simulink model "Abraham_PartC1"  (Simulink 9.1)
settings: Solver=VariableStepAuto  StartTime=0.0  StopTime=2  RelTol=1e-3
settings Model: Creator=sophi  LastModifiedBy=sophi
settings SolverCC: ZeroCrossAlgorithm=Adaptive
settings DataIOCC: SaveFormat=Dataset
settings OptimizationCC: LifeSpan=auto
settings DebuggingCC: UnderspecifiedInitializationDetection=Simplified  MergeDetectMultiDrivingBlocksExec=error  MaxConsecutiveZCsMsg=none  SFUnexpectedBacktrackingDiag=error  SFNoUnconditionalDefaultTransitionDiag=error  SFExecutionAtInitializationDiag=warning
settings HardwareCC: ProdBitPerPointer=64  ProdBitPerSizeT=64  ProdBitPerPtrDiffT=64  ProdLargestAtomicFloat=Float  ProdIntDivRoundTo=Zero  ProdEndianess=LittleEndian  ProdWordSize=64  ProdHWDeviceType=Intel->x86-64 (Windows64)
settings ModelReferenceCC: PropagateSignalLabelsOutOfModel=on
settings CodeAppCC: StateflowObjectComments=off
settings GRTTargetCC: TargetLangStandard=C99 (ISO)  CombineOutputUpdateFcns=on  GRTInterface=off
settings ConfigComp: CovMetricSettings=dwe  CovHtmlReporting=off  CovSaveCumulativeToWorkspaceVar=off  CovSaveSingleToWorkspaceVar=off  CovExternalEMLEnable=on

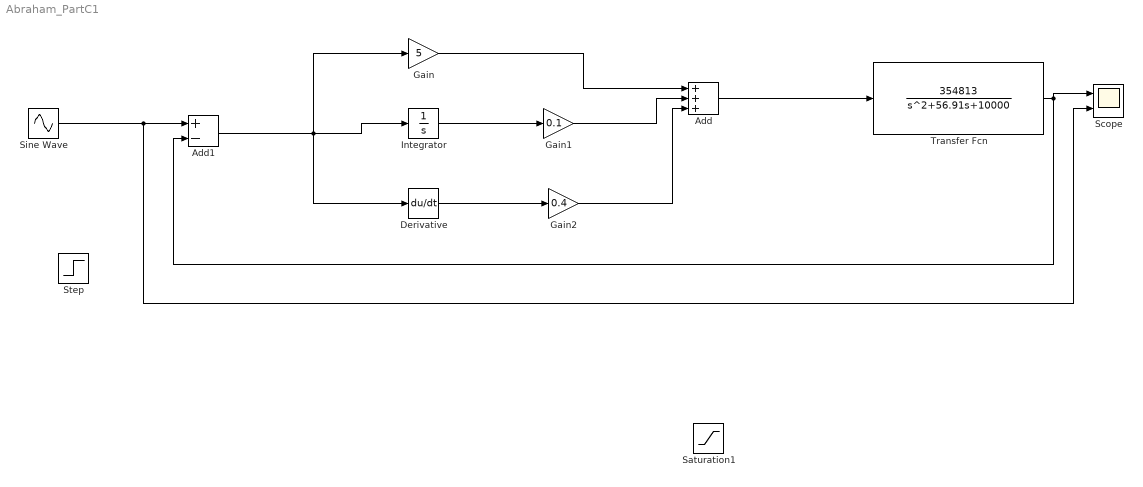
== system Abraham_PartC1 ==
  Add : Sum  Inputs=+++
  Add1 : Sum  Inputs=+-
  Derivative : Derivative
  Gain : Gain  Gain=5
  Gain1 : Gain  Gain=0.1
  Gain2 : Gain  Gain=0.4
  Integrator : Integrator
  Saturation1 : Saturate  UpperLimit=0.14  LowerLimit=-0.14
  Scope : Scope  NumInputPorts=2
  Sine Wave : Sin  Frequency=100  SampleTime=0
  Step : Step  After=5  SampleTime=0
  Transfer Fcn : TransferFcn  Numerator=[354813]  Denominator=[1 56.91 10000]
  wires:
  Integrator/1 -> Gain1/1
  Derivative/1 -> Gain2/1
  Gain/1 -> Add/1
  Gain1/1 -> Add/2
  Gain2/1 -> Add/3
  Transfer Fcn/1 -> Add1/2, Scope/1
  Sine Wave/1 -> Scope/2, Add1/1
  Add1/1 -> Integrator/1, Gain/1, Derivative/1
  Add/1 -> Transfer Fcn/1
